simulink model "block_pen_linear"  (R2018a)
settings: Solver=VariableStepAuto  StartTime=0.0  StopTime=10.0  RelTol=1e-3
values from neighbouring files (symbols this model uses):
  A = subs(A, ssx(i), ssx_Equilibrium_point(i))    [Drone_Linearization.m]    (also in Drone_SysId_2step.m = subs(A, v_syms(i), v_vals(i)); Drone_System.m = subs(A, v_syms(i), v_vals(i)); Drone_System_control.m = subs(A, v_syms(i), v_vals(i)); Drone_System_full.m = subs(A, v_syms(i), v_vals(i)))
  B = subs(B, ssx(i), ssx_Equilibrium_point(i))    [Drone_Linearization.m]    (also in Drone_SysId_2step.m = subs(B, v_syms(i), v_vals(i)); Drone_System.m = subs(B, v_syms(i), v_vals(i)); Drone_System_control.m = subs(B, v_syms(i), v_vals(i)); Drone_System_full.m = subs(B, v_syms(i), v_vals(i)))
  C = Gamma(1:p,1:size(A,1))    [SI_Ho_Kalman.m]    (also in SI_MOESP.m = Ok(1:p, 1:n); SI_N4SID.m = res(1+n:end, 1:n); SVD_identification.m; pen_SI.m = [1 0 0 0)
  ts = 0.001    [Drone_System.m]    (also in Drone_System_full.m; pen_SI.m = 0.02; pen_SI_close.m; pen_SI_open.m)
settings Model: Creator=ros  LastModifiedBy=ros

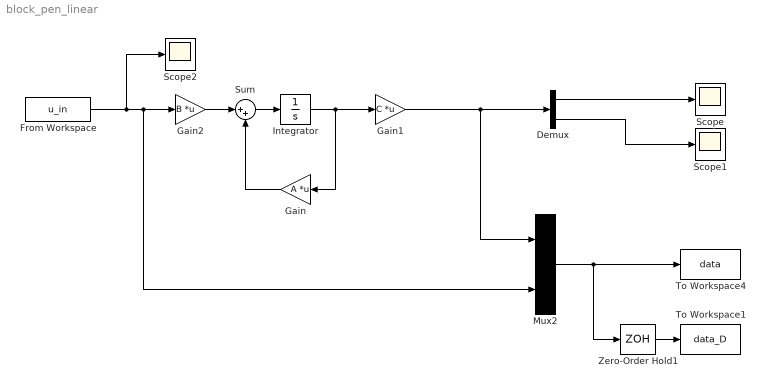
== system block_pen_linear ==
  Demux : Demux  Outputs=2
  From Workspace : FromWorkspace  VariableName=u_in  SampleTime=0.001
  Gain : Gain  Gain=A  Multiplication=Matrix(K*u)
  Gain1 : Gain  Gain=C  Multiplication=Matrix(K*u)
  Gain2 : Gain  Gain=B  Multiplication=Matrix(K*u)
  Integrator : Integrator
  Mux2 : Mux  Inputs=2
  Scope : Scope
  Scope1 : Scope
  Scope2 : Scope
  Sum : Sum  Inputs=|++
  To Workspace1 : ToWorkspace  VariableName=data_D  SaveFormat=Timeseries  SampleTime=-1
  To Workspace4 : ToWorkspace  VariableName=data  SaveFormat=Timeseries  SampleTime=-1
  Zero-Order Hold1 : ZeroOrderHold  SampleTime=ts
  wires:
  Integrator/1 -> Gain1/1, Gain/1
  Gain/1 -> Sum/2
  Gain2/1 -> Sum/1
  Sum/1 -> Integrator/1
  From Workspace/1 -> Scope2/1, Mux2/2, Gain2/1
  Gain1/1 -> Mux2/1, Demux/1
  Mux2/1 -> Zero-Order Hold1/1, To Workspace4/1
  Zero-Order Hold1/1 -> To Workspace1/1
  Demux/1 -> Scope/1
  Demux/2 -> Scope1/1
